simulink model "first"  (R2021b)
settings: Solver=ode2  StartTime=0.0  StopTime=766  FixedStep=0.1  MaxStep=0.2  MinStep=1e-20  RelTol=1e-3
values from neighbouring files (symbols this model uses):
  eng_map = [1009.3 1183.18 1588.89 1936.6 2318.13 2612.71 3371.09 3685.23 4014 7.66423 12.7737 24.635 ... (27 elements, 9x3)]    [eng_map.mat]
  hwfet = [0 1 2 3 4 5 6 7 8 9 10 11 ... (1532 elements, 766x2)]    [hwfet.mat]
undefined symbols (not defined in the file or in its folder): A_F, C_0, C_D, E_ess_max, eta_ess, g, G_diff, G_elec, grams_per_hr_to_gal_per_s, M_veh, meters_to_mi, mi_per_hr_to_m_per_s, param, r_wheel, rho, SOC_init
settings Model: Creator=wasynczu  LastModifiedBy=Kumar Chakravarthy
settings SolverCC: AlgebraicLoopSolver=TrustRegion
settings DebuggingCC: SFMachineParentedDataDiag=warning

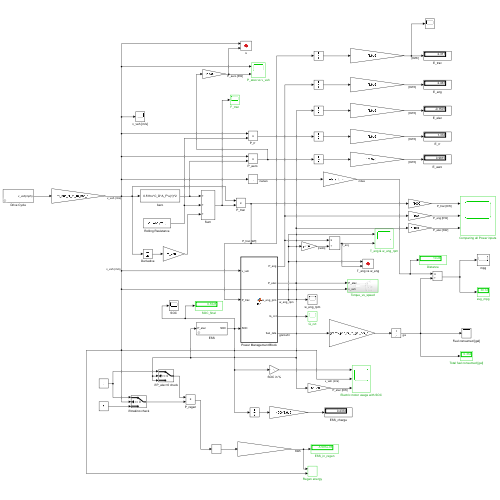
[thumbnail: Simulink's stored preview of the top-level diagram]
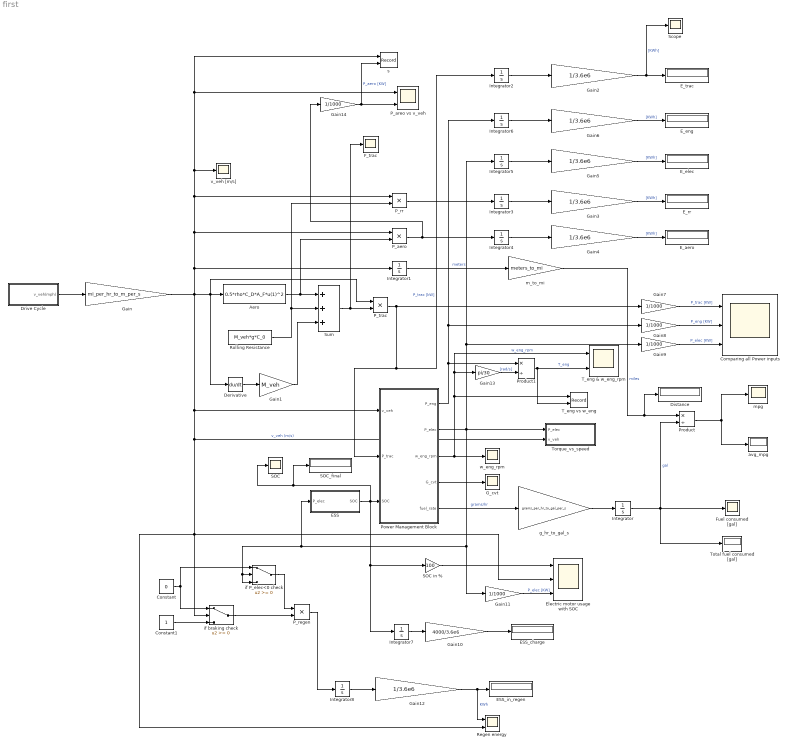
== system first ==
  Aero : Fcn  Expr=0.5*rho*C_D*A_F*u(1)^2
  Comparing all Power inputs : Scope  NumInputPorts=3
  Constant : Constant  Value=0
  Constant1 : Constant
  Derivative : Derivative
  Distance : Display
  Drive Cycle : Subsystem  mask{schedule=hwfet}
      mask prompts: schedule "drive schedule"
      mask init:
      | N=length(schedule(:,1));
  ESS : Subsystem  mask{E_max=E_ess_max, eta_ess=eta_ess}
      mask prompts: E_max "Maximum energy, J"; eta_ess "round-trip efficiency"
  ESS_charge : Display
  ESS_in_regen : Display
  E_aero : Display
  E_elec : Display
  E_eng : Display
  E_rr : Display
  E_trac : Display
  Electric motor usage with SOC : Scope  NumInputPorts=3
  F_trac : Scope
  Fuel consumed [gal] : Scope
  G_cvt : Scope
  Gain : Gain  Gain=mi_per_hr_to_m_per_s
  Gain1 : Gain  Gain=M_veh
  Gain10 : Gain  Gain=4000/3.6e6
  Gain{7..9,11,14} (5 alike) : Gain  Gain=1/1000
  Gain{2..6,12} (6 alike) : Gain  Gain=1/3.6e6
  Gain13 : Gain  Gain=pi/30
  Integrator{,1..8} (9 alike) : Integrator
  "P_aero " : Product
  P_areo vs v_veh : Scope  NumInputPorts=2
  P_regen : Product
  "P_rr " : Product
  P_trac : Product
  Power Management Block : MATLAB Function  TreatAsAtomicUnit=on
  Product : Product  Inputs=*/
  Product1 : Product  Inputs=*/
  Regen energy : Scope  NumInputPorts=2
  Rolling Resistance : Constant  Value=M_veh*g*C_0
  SOC : Scope
  SOC in % : Gain  Gain=100
  SOC_final : Display
  Scope : Scope
  Sum : Sum  Inputs=+++
  T_eng & w_eng_rpm : Scope  NumInputPorts=2
  T_eng vs w_eng : Record  FileSettingsInternal="{\"entries\":[{\"content\":{\"excelSettings\":{\"content\":{},\"type\":\"Streamout.ExcelSettings\"}},\"type\":\"Streamout.FileSettingStorage\",\"uuid\":\"e8810c02-a781-440f-a0aa-6ea0337eb554\"}],\"packageUris\":[\"http://schema.mathworks.com/mf0/streamout_blocks/R2020a\"],\"version\":\"1.0\"}"  Layout=[1 1]  SignalsInternal="{\"entries\":[{\"content\":{\"signals\":[{\"content\":{\"blockPath\":[\"first/T_eng vs w_eng\"],\"channel\":[],\"dimensions\":[1],\"domain\":\"first/T_eng vs w_eng\",\"lineColor\":\"#a2142f\",\"plots\":[],\"port\":1,\"sid\":[\"\"],\"signalID\":353,\"signalName\":\"w_eng_rpm\"},\"type\":\"RecordBlkView.Signal\",\"uuid\":\"3905639b-b552-46c2-b388-1891f00bc392\"},{\"content\":{\"blockPath\":[\"first/T_eng vs w_eng\"],\"channel\":[],\"dimensions\":[1],\"domain\":\"first/T_eng vs w_eng\",\"lineColor\":\"#139fff\",\"plots\":[],\"port\":2,\"sid\":[\"\"],\"signalID\":357,\"signalName\":\"T_eng\"},\"type\":\"RecordBlkView.Signal\",\"uuid\":\"46e10628-2ee3-409f-94e9-c2aadcdcf48a\"}]},\"type\":\"RecordBlkView.InputSignals\",\"uuid\":\"a575c4f8-c719-4be2-8917-6ef6ebe34d3e\"}],\"packageUris\":[\"http://schema.mathworks.com/mf0/streamout_blocks/R2020a\"],\"version\":\"1.0\"}"  VisualizationBindings="{\"xyplotplugin\":{\"info\":[{\"series\":[],\"subplotID\":1}]}}"  CompatibilityTag=XY
  Torque_vs_speed : Subsystem
  Total fuel consumed [gal] : Display
  avg_mpg : Display
  g_hr_to_gal_s : Gain  Gain=grams_per_hr_to_gal_per_s
  if P_elec<0 check : Switch  OutDataTypeStr=double
  if braking check : Switch  OutDataTypeStr=double
  m_to_mi : Gain  Gain=meters_to_mi
  mpg : Scope
  s : Record  FileSettingsInternal="{\"entries\":[{\"content\":{\"excelSettings\":{\"content\":{},\"type\":\"Streamout.ExcelSettings\"}},\"type\":\"Streamout.FileSettingStorage\",\"uuid\":\"82f50792-d557-49ae-9ff4-48ee91707643\"}],\"packageUris\":[\"http://schema.mathworks.com/mf0/streamout_blocks/R2020a\"],\"version\":\"1.0\"}"  Layout=[1 1]  SignalsInternal="{\"entries\":[{\"content\":{\"signals\":[{\"content\":{\"blockPath\":[\"first/s\"],\"channel\":[],\"dimensions\":[1],\"domain\":\"first/s\",\"lineColor\":\"#64d413\",\"plots\":[],\"port\":1,\"sid\":[\"\"],\"signalID\":369,\"signalName\":\"v_veh (m/s)\"},\"type\":\"RecordBlkView.Signal\",\"uuid\":\"3b5b11c4-51da-4adc-b968-fa1dcc70d426\"},{\"content\":{\"blockPath\":[\"first/s\"],\"channel\":[],\"dimensions\":[1],\"domain\":\"first/s\",\"lineColor\":\"#ff13a6\",\"plots\":[],\"port\":2,\"sid\":[\"\"],\"signalID\":373,\"signalName\":\"P_aero [KW]\"},\"type\":\"RecordBlkView.Signal\",\"uuid\":\"d1f209af-cd75-44ae-8053-2c5e7dc65aef\"}]},\"type\":\"RecordBlkView.InputSignals\",\"uuid\":\"26f492a8-61b9-4492-86e3-164c0d2a7e81\"}],\"packageUris\":[\"http://schema.mathworks.com/mf0/streamout_blocks/R2020a\"],\"version\":\"1.0\"}"  VisualizationBindings="{\"xyplotplugin\":{\"info\":[{\"series\":[],\"subplotID\":1}]}}"  CompatibilityTag=XY
  v_veh [m/s] : Scope
  w_eng_rpm : Scope
  wires:
  Drive Cycle/1(v_veh(mph)) -> Gain/1
  Gain/1 -> "P_aero "/1, "P_rr "/1, s/1, P_areo vs v_veh/1, v_veh [m/s]/1, Integrator1/1, Torque_vs_speed/2(v_veh), Electric motor usage with SOC/2, Regen energy/2, if braking check/2, Power Management Block/1(v_veh), P_trac/1, Aero/1, Derivative/1  "v_veh (m/s)"
  Aero/1 -> "P_aero "/2, Sum/1
  Rolling Resistance/1 -> "P_rr "/2, Sum/2
  Derivative/1 -> Gain1/1
  Sum/1 -> F_trac/1, P_trac/2
  Gain1/1 -> Sum/3
  ESS/1(SOC) -> Integrator7/1, SOC in %/1, SOC_final/1, SOC/1, Power Management Block/3(SOC)
  Power Management Block/2(P_elec) -> Integrator5/1, Gain9/1, Gain11/1, if P_elec<0 check/3, if P_elec<0 check/2, ESS/1(P_elec), Torque_vs_speed/1(P_elec)
  Power Management Block/5(fuel_rate) -> g_hr_to_gal_s/1  "grams/hr"
  g_hr_to_gal_s/1 -> Integrator/1
  Integrator1/1 -> m_to_mi/1  "meters"
  Integrator/1 -> Fuel consumed [gal]/1, Total fuel consumed [gal]/1, Product/2  "gal"
  m_to_mi/1 -> Distance/1, Product/1  "miles"
  Product/1 -> avg_mpg/1, mpg/1
  Power Management Block/1(P_eng) -> Integrator6/1, Gain8/1, Product1/1
  Power Management Block/3(w_eng_rpm) -> T_eng vs w_eng/1, T_eng & w_eng_rpm/1, Gain13/1, w_eng_rpm/1  "w_eng_rpm"
  Power Management Block/4(G_cvt) -> G_cvt/1
  "P_rr "/1 -> Integrator3/1
  "P_aero "/1 -> Gain14/1, Integrator4/1
  Integrator3/1 -> Gain3/1
  Integrator4/1 -> Gain4/1
  Gain4/1 -> E_aero/1  "[KWh]"
  Gain3/1 -> E_rr/1  "[KWh]"
  Gain5/1 -> E_elec/1  "[KWh]"
  Integrator5/1 -> Gain5/1
  Gain6/1 -> E_eng/1  "[KWh]"
  Integrator6/1 -> Gain6/1
  Gain2/1 -> Scope/1, E_trac/1  "[KWh]"
  Integrator2/1 -> Gain2/1
  SOC in %/1 -> Electric motor usage with SOC/1
  Gain7/1 -> Comparing all Power inputs/1  "P_trac [KW]"
  Gain8/1 -> Comparing all Power inputs/2  "P_eng [KW]"
  Gain9/1 -> Comparing all Power inputs/3  "P_elec [KW]"
  Integrator7/1 -> Gain10/1
  Gain10/1 -> ESS_charge/1
  Gain11/1 -> Electric motor usage with SOC/3  "P_elec [KW]"
  Constant/1 -> if braking check/1, if P_elec<0 check/1
  Constant1/1 -> if braking check/3
  if P_elec<0 check/1 -> P_regen/1
  if braking check/1 -> P_regen/2
  Integrator8/1 -> Gain12/1
  Gain12/1 -> Regen energy/1, ESS_in_regen/1  "KWh"
  P_regen/1 -> Integrator8/1
  Product1/1 -> T_eng vs w_eng/2, T_eng & w_eng_rpm/2  "T_eng"
  Gain13/1 -> Product1/2  "[rad/s]"
  Gain14/1 -> s/2, P_areo vs v_veh/2  "P_aero [KW]"
  P_trac/1 -> Gain7/1, Integrator2/1, Power Management Block/2(P_trac)  "P_trac [kW]"

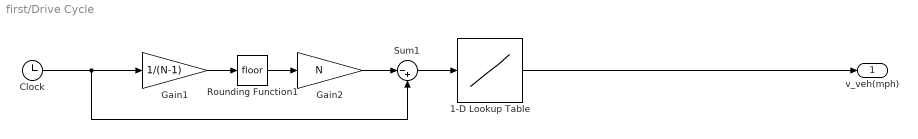
== system first/Drive Cycle ==
  1-D Lookup Table : Lookup_n-D  NumberOfTableDimensions=1  BreakpointsForDimension1=schedule(:,1)  Table=schedule(:,2)  InterpMethod=Cubic spline  InternalRulePriority=Speed  RndMeth=Simplest  InputSameDT=on
  Clock : Clock
  Gain1 : Gain  Gain=1/(N-1)
  Gain2 : Gain  Gain=N
  Rounding Function1 : Rounding
  Sum1 : Sum  Inputs=|-+
  v_veh(mph) : Outport  VectorParamsAs1DForOutWhenUnconnected=off
  wires:
  Clock/1 -> Gain1/1, Sum1/2
  Sum1/1 -> 1-D Lookup Table/1
  Gain2/1 -> Sum1/1
  Rounding Function1/1 -> Gain2/1
  Gain1/1 -> Rounding Function1/1
  1-D Lookup Table/1 -> v_veh(mph)/1

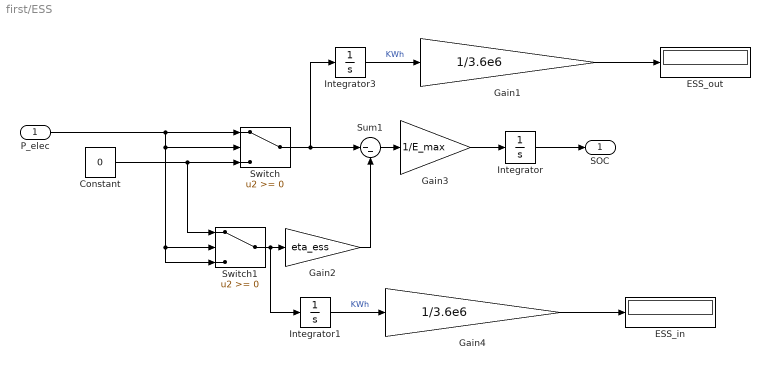
== system first/ESS ==
  P_elec : Inport
  Constant : Constant  Value=0
  ESS_in : Display
  ESS_out : Display
  Gain1 : Gain  Gain=1/3.6e6
  Gain2 : Gain  Gain=eta_ess
  Gain3 : Gain  Gain=1/E_max  OutDataTypeStr=fixdt('double', 'DataTypeOverride', 'Off')
  Gain4 : Gain  Gain=1/3.6e6
  Integrator : Integrator  InitialCondition=SOC_init  LimitOutput=on  UpperSaturationLimit=1  LowerSaturationLimit=0
  Integrator1 : Integrator
  Integrator3 : Integrator
  Sum1 : Sum  Inputs=|--
  Switch : Switch  OutDataTypeStr=double
  Switch1 : Switch  OutDataTypeStr=double
  SOC : Outport  VectorParamsAs1DForOutWhenUnconnected=off
  wires:
  P_elec/1 -> Switch1/2, Switch1/3, Switch/2, Switch/1
  Gain3/1 -> Integrator/1
  Gain2/1 -> Sum1/2
  Switch1/1 -> Integrator1/1, Gain2/1
  Sum1/1 -> Gain3/1
  Switch/1 -> Integrator3/1, Sum1/1
  Constant/1 -> Switch1/1, Switch/3
  Integrator/1 -> SOC/1
  Gain1/1 -> ESS_out/1
  Integrator3/1 -> Gain1/1  "KWh"
  Gain4/1 -> ESS_in/1
  Integrator1/1 -> Gain4/1  "KWh"

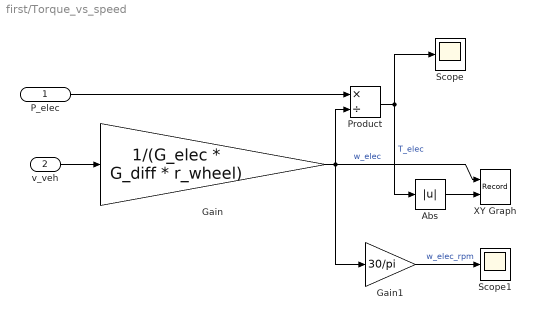
== system first/Torque_vs_speed ==
  P_elec : Inport
  v_veh : Inport  Port=2
  Abs : Abs
  Gain : Gain  Gain=1/(G_elec * G_diff * r_wheel)
  Gain1 : Gain  Gain=30/pi
  Product : Product  Inputs=*/
  Scope : Scope
  Scope1 : Scope
  XY Graph : Record  FileSettingsInternal="{\"entries\":[{\"content\":{\"excelSettings\":{\"content\":{},\"type\":\"Streamout.ExcelSettings\"}},\"type\":\"Streamout.FileSettingStorage\",\"uuid\":\"02627308-9a79-425d-aeec-e9e94ddd7ae0\"}],\"packageUris\":[\"http://schema.mathworks.com/mf0/streamout_blocks/R2020a\"],\"version\":\"1.0\"}"  Layout=[1 1]  SignalsInternal="{\"entries\":[{\"content\":{\"signals\":[{\"content\":{\"blockPath\":[\"first/Torque_vs_speed/XY Graph\"],\"channel\":[],\"dimensions\":[1],\"domain\":\"first/Torque_vs_speed/XY Graph\",\"lineColor\":\"#a2142f\",\"plots\":[1],\"port\":1,\"sid\":[\"\"],\"signalID\":361,\"signalName\":\"w_elec\"},\"type\":\"RecordBlkView.Signal\",\"uuid\":\"d0663536-23cd-4689-8d14-dfc1729d4cf1\"},{\"content\":{\"blockPath\":[\"first/Torque_vs_speed/XY Graph\"],\"channel\":[],\"dimensions\":[1],\"domain\":\"first/Torque_vs_speed/XY Graph\",\"lineColor\":\"#139fff\",\"plots\":[1],\"port\":2,\"sid\":[\"\"],\"signalID\":365,\"signalName\":\"Abs\"},\"type\":\"RecordBlkView.Signal\",\"uuid\":\"b5d84633-54d2-4fe4-87ac-75b093820aad\"}]},\"type\":\"RecordBlkView.InputSignals\",\"uuid\":\"090edd6d-f316-49f3-9067-15d37f97f172\"}],\"packageUris\":[\"http://schema.mathworks.com/mf0/streamout_blocks/R2020a\"],\"version\":\"1.0\"}"  VisualizationBindings="{\"xyplotplugin\":{\"info\":[{\"series\":[{\"bindingParametersList\":[{\"parameter\":\"X-Axis\",\"signalID\":361,\"signalName\":\"w_elec\"},{\"parameter\":\"Y-Axis\",\"signalID\":365,\"signalName\":\"Abs\"}],\"seriesID\":10917}],\"subplotID\":1}]}}"  CompatibilityTag=XY  st=-1
  wires:
  P_elec/1 -> Product/1
  Product/1 -> Scope/1, Abs/1  "T_elec"
  v_veh/1 -> Gain/1
  Gain/1 -> Gain1/1, XY Graph/1, Product/2  "w_elec"
  Abs/1 -> XY Graph/2
  Gain1/1 -> Scope1/1  "w_elec_rpm"

== matlab function first/Power Management Block ==
  data: v_veh input; P_eng output; P_trac input; SOC input; P_elec output; w_eng_rpm output; G_cvt output; fuel_rate output; param parameter; eng_map parameter
function [P_eng, P_elec, w_eng_rpm, G_cvt, fuel_rate] = fcn(v_veh, P_trac, SOC, param, eng_map)
%#codegen
%inputs:
    % v_veh, m/s
    % P_trac, W
    % SOC
    % param, structure of parameters
    % eng_map

% outputs:
    %   P_gen, P_elec in W
    %   w_eng_rpm, rpm
    %   G_cvt (cvt ratio)
    %   Fuel rate, grams/hr

v_veh_min = param.v_veh_min;    % minimum vehicle speed for engine to stay engaged, in m/s
P_eng_min = param.P_eng_min;    % minimum engine power in W
P_eng_max = param.P_eng_max ;   % maximum engine power
G_cvt_min = param.G_cvt_min;    % minimum cvt  ratio
G_diff = param.G_diff;          % differential gear ratio
r_wheel = param.r_wheel;        % wheel radius in m

if (v_veh < v_veh_min)  % disengage clutch, idle engine, electric propulsion
   P_elec = P_trac;
   P_eng = 0;
   fuel_rate = 0; % g/hr;
   w_eng_rpm = 1000; % rpm
   G_cvt = G_cvt_min;
   return  
end

% if here, v_veh > v_veh_min
if(P_trac < P_eng_min)   % clutch engaged but engine idling
   P_elec = P_trac;
   fuel_rate = 0;
   P_eng = 0;
   w_eng_rpm =  1000; % rpm
   w_eng = w_eng_rpm * pi / 30; % rad/s
   % set G_cvt so engine speed is 1000 rpm
   G_cvt = v_veh/G_diff/w_eng/r_wheel;
   return     
end

if(P_trac > P_eng_max) % high-speed boost
   P_elec = P_trac - P_eng_max;
   P_eng = P_eng_max;
   bsfc = interp1(eng_map(:,2), eng_map(:,3), P_eng/1000, 'pchip', 'extrap');
   fuel_rate = bsfc*P_eng/1000; % grams/hr
   w_eng_rpm = interp1(eng_map(:,2), eng_map(:,1), P_eng/1000, 'pchip', 'extrap');
   w_eng = w_eng_rpm * pi / 30; % convert to rad/s
   G_cvt =  v_veh/r_wheel/G_diff/w_eng; % required CVT ratio
   return   
end

% if here, v_veh > v_veh_min and P_eng_min < P_trac < P_eng_max
% try to get SOC back to 0.5

%P_elec = 4000*sign(SOC - 0.5); 
P_elec = 20000*(SOC - 0.5); 
if(P_elec > 4000) 
    P_elec = 4000; 
end
if(P_elec < -4000) 
    P_elec = -4000;
end

P_eng = P_trac - P_elec;


if(P_eng < P_eng_min) 
   % clutch engaged, but no fuel
   P_eng = 0;
   P_elec = P_trac;
   fuel_rate = 0;
   w_eng_rpm = 1000;
   w_eng = w_eng_rpm * 2 * pi / 60; % in rad/s
   % set G_cvt so engine speed is 1000 rpm
   G_cvt = v_veh/G_diff/w_eng/r_wheel;
   return
end

if(P_eng > P_eng_max)
    P_eng = P_eng_max;
    P_elec = P_trac - P_eng_max;
end

bsfc = interp1(eng_map(:,2), eng_map(:,3), P_eng/1000, 'pchip', 'extrap');
fuel_rate = bsfc*P_eng/1000; % grams/hr

w_eng_rpm = interp1(eng_map(:,2), eng_map(:,1), P_eng/1000, 'pchip', 'extrap');
if(w_eng_rpm < 1000)
    w_eng_rpm = 1000;
end
w_eng = w_eng_rpm * pi / 30;  % convert to rad/s
G_cvt =  v_veh/r_wheel/G_diff/w_eng;

if (G_cvt < G_cvt_min) % set G_cvt = G_cvt_min, recalculate w_eng, P_eng, and P_elec
   G_cvt = G_cvt_min;
   w_eng = v_veh/G_diff/r_wheel/G_cvt;
   w_eng_rpm = w_eng*30/pi;  % in rpm
   P_eng = 1000*interp1(eng_map(:,1), eng_map(:,2), w_eng_rpm, 'pchip', 'extrap'); % in W
   if(P_eng < 0)
       P_eng = 0;
   end
   P_elec = P_trac - P_eng;
   bsfc = interp1(eng_map(:,1), eng_map(:,3), w_eng_rpm, 'pchip', 'extrap');
   fuel_rate = bsfc*P_eng/1000; % grams/hr
 end
